simulink model "es601_ex04s"  (R2019a)
settings: Solver=FixedStepAuto  StartTime=0.0  StopTime=10  FixedStep=0.05  RelTol=1e-3
settings Model: Creator=Admin-PC  LastModifiedBy=Admin-PC

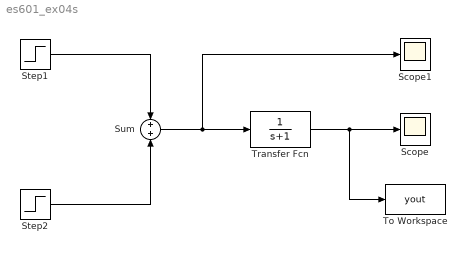
== system es601_ex04s ==
  Scope : Scope
  Scope1 : Scope
  Step1 : Step  Time=0  After=10  SampleTime=0
  Step2 : Step  Time=3  After=-10  SampleTime=0
  Sum : Sum
  To Workspace : ToWorkspace  VariableName=yout  SampleTime=-1
  Transfer Fcn : TransferFcn  Denominator=[1 1]
  wires:
  Sum/1 -> Scope1/1, Transfer Fcn/1
  Transfer Fcn/1 -> To Workspace/1, Scope/1
  Step2/1 -> Sum/2
  Step1/1 -> Sum/1
